simulink model "elevator"  (R2018b)
settings: Solver=VariableStepAuto  StartTime=0.0  StopTime=10.0  RelTol=1e-3
settings Model: Creator=Sjoerd  LastModifiedBy=Sjoerd

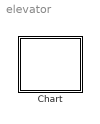
== system elevator ==
  Chart : Stateflow chart  TreatAsAtomicUnit=on

== stateflow chart elevator/Chart ==
  state Doors
    state Open
    state Closed
    (default) -> Open
    Closed -> Open
    Open -> Closed
  state Button1
    state NotPressed
    state Pressed
    (default) -> NotPressed
    Pressed -> NotPressed
    NotPressed -> Pressed
  (default) -> Doors
